simulink model "cascadefilter"  (R2020b)
settings: Solver=VariableStepAuto  StartTime=0.0  StopTime=10.0  RelTol=1e-3
settings Model: Creator=shivanshu shukla  LastModifiedBy=shivanshu shukla

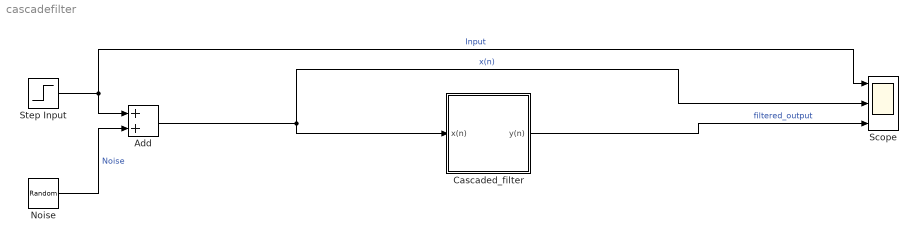
== system cascadefilter ==
  Add : Sum
  Cascaded_filter : Subsystem
  Noise : RandomNumber  SampleTime=0.1
  Scope : Scope  NumInputPorts=3
  Step Input : Step  SampleTime=0
  wires:
  Add/1 -> Scope/2, Cascaded_filter/1(x(n))  "x(n)"
  Cascaded_filter/1(y(n)) -> Scope/3  "filtered_output"
  Step Input/1 -> Add/1, Scope/1  "Input"
  Noise/1 -> Add/2  "Noise"

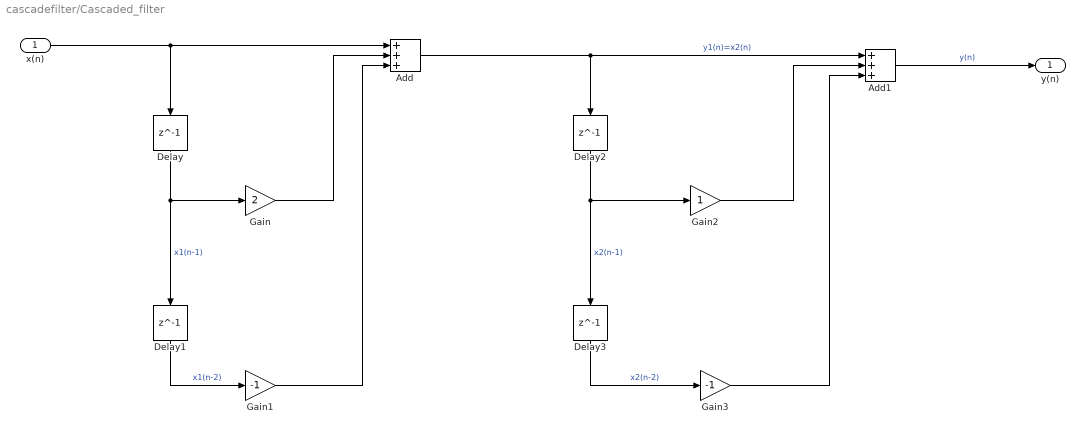
== system cascadefilter/Cascaded_filter ==
  x(n) : Inport
  Add : Sum  Inputs=+++
  Add1 : Sum  Inputs=+++
  Delay{,1..3} (4 alike) : Delay  DelayLength=1
  Gain : Gain  Gain=2
  Gain1 : Gain  Gain=-1
  Gain2 : Gain
  Gain3 : Gain  Gain=-1
  y(n) : Outport
  wires:
  Add/1 -> Add1/1, Delay2/1  "y1(n)=x2(n)"
  x(n)/1 -> Add/1, Delay/1
  Delay/1 -> Delay1/1, Gain/1  "x1(n-1)"
  Gain3/1 -> Add1/3
  Add1/1 -> y(n)/1  "y(n)"
  Delay1/1 -> Gain1/1  "x1(n-2)"
  Gain2/1 -> Add1/2
  Delay2/1 -> Gain2/1, Delay3/1  "x2(n-1)"
  Gain/1 -> Add/2
  Delay3/1 -> Gain3/1  "x2(n-2)"
  Gain1/1 -> Add/3
